simulink model "pwm_oora_emaatha"  (R2013a)
settings: Solver=ode45  StartTime=0.0  StopTime=inf  RelTol=1e-3
libraries: simulink x1
settings Model: Creator=user-pc  LastModifiedBy=user-pc

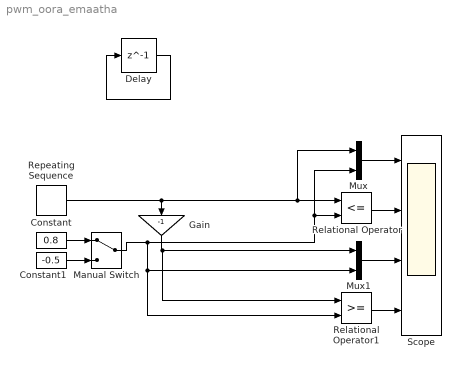
== system pwm_oora_emaatha ==
  Constant : Constant  Value=0.8
  Constant1 : Constant  Value=-0.5
  Delay : Delay  DelayLength=1  InitialCondition=0  SampleTime=0.00000001
  Gain : Gain  Gain=-1
  Manual Switch : ManualSwitch
  Mux : Mux  Inputs=2
  Mux1 : Mux  Inputs=2
  Relational Operator : RelationalOperator  Operator=<=  OutDataTypeStr=boolean
  Relational Operator1 : RelationalOperator  OutDataTypeStr=boolean
  Repeating Sequence : simulink/Sources/Repeating Sequence  rep_seq_t=[0 0.0005 0.0005 0.001]  rep_seq_y=[0 1 0 1]
  Scope : Scope  NumInputPorts=4
      settings: TickLabels=on  YMin=-0.6~-0.2~-1.2~-0.2  YMax=1.2~1.2~1~1.2
  wires:
  Constant/1 -> Manual Switch/1
  Constant1/1 -> Manual Switch/2
  Manual Switch/1 -> Relational Operator1/2, Mux1/2, Mux/2, Relational Operator/2
  Repeating Sequence/1 -> Mux/1, Relational Operator/1, Gain/1
  Relational Operator/1 -> Scope/2
  Delay/1 -> Delay/1
  Mux/1 -> Scope/1
  Relational Operator1/1 -> Scope/4
  Mux1/1 -> Scope/3
  Gain/1 -> Relational Operator1/1, Mux1/1
